simulink model "tarefa11"  (R2022b)
settings: Solver=VariableStepAuto  StartTime=0.0  StopTime=30.0  RelTol=1e-3
values from neighbouring files (symbols this model uses):
  d = -0.15    [lab11.m]
  F = [0.001 -0.382; 0.35 0.739]    [lab11.m]
  H = [0.35;0.239]    [lab11.m]
  K = place(F,H,polos_dominantes)    [lab11.m]
  R = 1.25    [lab11.m]
  td = 15    [lab11.m]
undefined symbols (not defined in the file or in its folder): Cd, T0
settings Model: Creator=hugo_  LastModifiedBy=hugo_

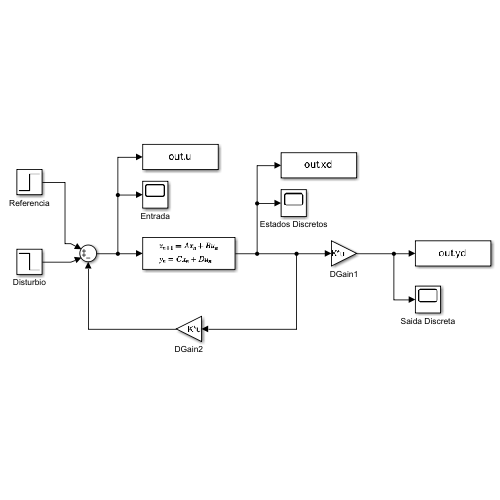
[thumbnail: Simulink's stored preview of the top-level diagram]
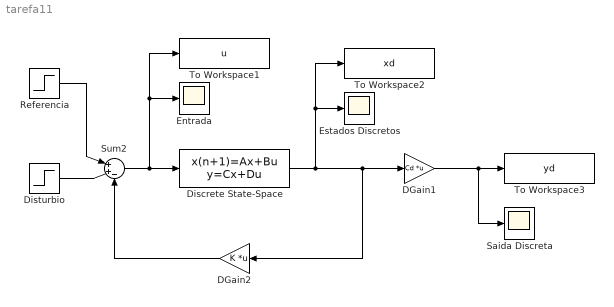
== system tarefa11 ==
  DGain1 : Gain  Gain=Cd  Multiplication=Matrix(K*u)
  DGain2 : Gain  Gain=K  Multiplication=Matrix(K*u)
  Discrete State-Space : DiscreteStateSpace  A=F  B=H  C=[1 0; 0 1]  D=[0;0]  SampleTime=T0
  Disturbio : Step  Time=td  After=d  SampleTime=0
  Entrada : Scope
  Estados Discretos : Scope
  Referencia : Step  Time=0  After=R  SampleTime=0
  Saida Discreta : Scope
  Sum2 : Sum  Inputs=|++-
  To Workspace1 : ToWorkspace  VariableName=u  SaveFormat=Timeseries  SampleTime=-1
  To Workspace2 : ToWorkspace  VariableName=xd  SaveFormat=Timeseries  SampleTime=-1
  To Workspace3 : ToWorkspace  VariableName=yd  SaveFormat=Timeseries  SampleTime=-1
  wires:
  Discrete State-Space/1 -> To Workspace2/1, Estados Discretos/1, DGain2/1, DGain1/1
  DGain1/1 -> Saida Discreta/1, To Workspace3/1
  Sum2/1 -> Entrada/1, To Workspace1/1, Discrete State-Space/1
  Referencia/1 -> Sum2/1
  Disturbio/1 -> Sum2/2
  DGain2/1 -> Sum2/3
